simulink model "sampleModel1"  (R2021a)
settings: Solver=VariableStepAuto  StartTime=0.0  StopTime=50  RelTol=1e-3
undefined symbols (not defined in the file): DiscIntNeverNeededParam, magnitude, Newton, Raphson
libraries: simulink x92, pid_lib x10
(part 2 of 5)

== system sampleModel1/cfblk99 ==
  cfblk1 : Inport
  cfblk11 : Inport  Port=2
  cfblk12 : Inport  Port=3
  cfblk13 : Inport  Port=4
  cfblk14 : Inport  Port=5
  Action Port : ActionPort  ActionPortLabel=else
  cfblk10 : Subsystem
  cfblk3 : simulink/Math Operations/Slider Gain  gain=1  low=0  high=2
  cfblk4 : Squeeze
  cfblk5 : Sqrt  Operator=rSqrt  AlgorithmType=Newton-Raphson  SaturateOnIntegerOverflow=on
  cfblk6 : Constant  Value=[-6555592.349522]  SampleTime=1
  cfblk7 : Constant  Value=[-863944611.741175]  SampleTime=1
  cfblk8 : Constant  Value=[-802487376.058000]  SampleTime=1
  cfblk9 : Subsystem
  cfblk2 : Outport
  cfblk15 : Outport  Port=2
  wires:
  cfblk11/1 -> cfblk4/1
  cfblk12/1 -> cfblk5/1
  cfblk7/1 -> cfblk15/1
  cfblk3/1 -> cfblk10/1(cfblk1), cfblk9/4(cfblk10)
  cfblk1/1 -> cfblk10/2(cfblk10)
  cfblk4/1 -> cfblk3/1
  cfblk6/1 -> cfblk10/3(cfblk11)
  cfblk8/1 -> cfblk2/1
  cfblk5/1 -> cfblk10/4(cfblk12)
  cfblk14/1 -> cfblk9/1(cfblk1)
  cfblk13/1 -> cfblk10/5(cfblk13)
  cfblk10/1(cfblk2) -> cfblk9/2(cfblk8)
  cfblk10/2(cfblk14) -> cfblk9/3(cfblk9)

== system sampleModel1/cfblk101/cfblk12 ==
  cfblk1 : Inport
  cfblk6 : Inport  Port=2
  cfblk7 : Inport  Port=3
  cfblk3 : Delay
  cfblk4 : Product  Inputs=*
  cfblk5 : Constant  Value=[722696352.833129]  SampleTime=1
  cfblk2 : Outport
  cfblk8 : Outport  Port=2
  wires:
  cfblk7/1 -> cfblk8/1
  cfblk1/1 -> cfblk4/1
  cfblk4/1 -> cfblk3/1
  cfblk6/1 -> cfblk2/1

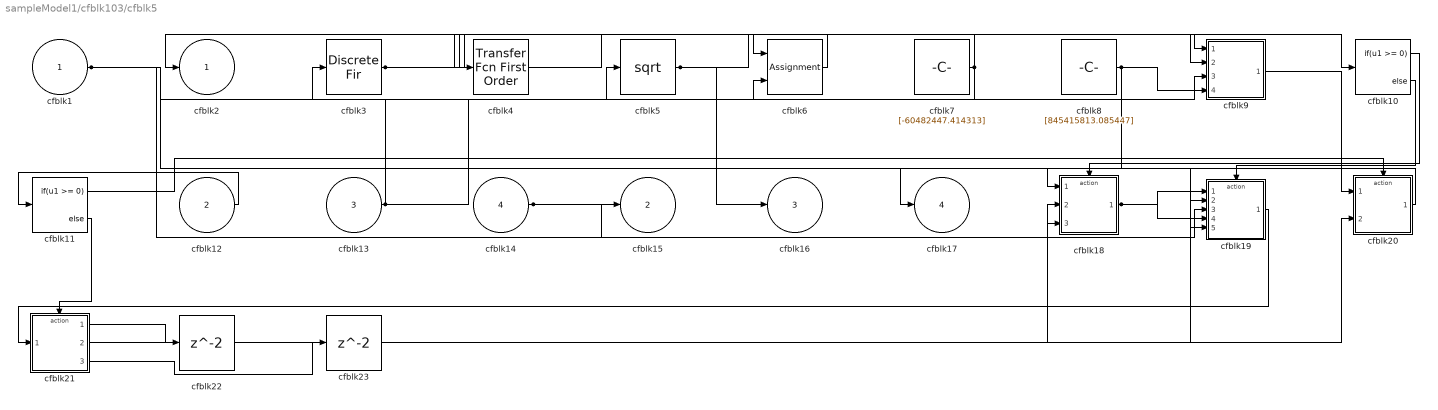
== system sampleModel1/cfblk103/cfblk5 ==
  cfblk1 : Inport
  cfblk12 : Inport  Port=2
  cfblk13 : Inport  Port=3
  cfblk14 : Inport  Port=4
  cfblk10 : If  IfExpression=u1 >= 0  SampleTime=1
  cfblk11 : If  IfExpression=u1 >= 0  SampleTime=1
  cfblk18 : Subsystem  TreatAsAtomicUnit=on
  cfblk19 : Subsystem  TreatAsAtomicUnit=on
  cfblk20 : Subsystem  TreatAsAtomicUnit=on
  cfblk21 : Subsystem  TreatAsAtomicUnit=on
  cfblk22 : Delay
  cfblk23 : Delay
  cfblk3 : DiscreteFir
  cfblk4 : simulink/Discrete/Transfer Fcn First Order  PoleZ=0.95  ICPrevOutput=0.0  DoSatur=off
  cfblk5 : Sqrt  SaturateOnIntegerOverflow=on
  cfblk6 : Assignment  DiagnosticForDimensions=Warning  IndexOptions=Index vector (dialog)  Indices=1  OutputSizes=1
  cfblk7 : Constant  Value=[-60482447.414313]  SampleTime=1
  cfblk8 : Constant  Value=[845415813.085447]  SampleTime=1
  cfblk9 : Subsystem
  cfblk2 : Outport
  cfblk15 : Outport  Port=2
  cfblk16 : Outport  Port=3
  cfblk17 : Outport  Port=4
  wires:
  cfblk20/1(cfblk2) -> cfblk17/1
  cfblk19/1(cfblk2) -> cfblk21/1(cfblk1)
  cfblk18/1(cfblk2) -> cfblk19/1(cfblk1), cfblk19/4(cfblk15)
  cfblk8/1 -> cfblk18/1(cfblk1), cfblk9/4(cfblk16)
  cfblk3/1 -> cfblk9/1(cfblk1), cfblk10/1
  cfblk14/1 -> cfblk15/1, cfblk19/3(cfblk14)
  cfblk13/1 -> cfblk5/1, cfblk3/1
  cfblk6/1 -> cfblk2/1
  cfblk4/1 -> cfblk6/1
  cfblk5/1 -> cfblk16/1, cfblk9/2(cfblk14)
  cfblk9/1(cfblk2) -> cfblk20/1(cfblk1)
  cfblk1/1 -> cfblk18/2(cfblk6), cfblk9/3(cfblk15), cfblk19/5(cfblk16)
  cfblk12/1 -> cfblk11/1
  cfblk21/2(cfblk14) -> cfblk20/2(cfblk11)
  cfblk7/1 -> cfblk4/1, cfblk6/2
  cfblk10/1 -> cfblk18/Action
  cfblk10/2 -> cfblk19/Action
  cfblk11/1 -> cfblk20/Action
  cfblk11/2 -> cfblk21/Action
  cfblk21/1(cfblk2) -> cfblk22/1
  cfblk22/1 -> cfblk19/2(cfblk13)
  cfblk21/3(cfblk15) -> cfblk23/1
  cfblk23/1 -> cfblk18/3(cfblk7)

== system sampleModel1/cfblk104/cfblk18 ==
  cfblk1 : Inport
  cfblk6 : Inport  Port=2
  cfblk7 : Inport  Port=3
  cfblk8 : Inport  Port=4
  Action Port : ActionPort  ActionPortLabel=if(u1 >= 0)
  cfblk10 : Subsystem  TreatAsAtomicUnit=on
  cfblk11 : Delay
  cfblk12 : Delay
  cfblk3 : pid_lib/PID Controller (2DOF)  Controller=PID  Form=Parallel  TimeDomain=Discrete-time  UseExternalTs=off  SampleTime=-1  IntegratorMethod=Forward Euler  FilterMethod=Forward Euler  ControllerParametersSource=internal  P=1  I=1  D=0  UseFilter=on  N=100  b=1  c=1  TunerSelectOption=Transfer Function Based (PID Tuner App)  InitialConditionSource=internal  InitialConditionForIntegrator=0  InitialConditionForFilter=0  DifferentiatorICPrevScaledInput=0  ExternalReset=none  TrackingMode=off  Kt=1  LimitOutput=off  SatLimitsSource=internal  UpperSaturationLimit=inf  LowerSaturationLimit=-inf  LinearizeAsGain=off  AntiWindupMode=none  Kb=1  POutMin=[]  POutMax=[]  IOutMin=[]  IOutMax=[]  DOutMin=[]  DOutMax=[]  NOutMin=[]  NOutMax=[]  bOutMin=[]  bOutMax=[]  cOutMin=[]  cOutMax=[]  SumOutMin=[]  SumOutMax=[]  SaturationOutMin=[]  SaturationOutMax=[]  PParamMin=[]  PParamMax=[]  IParamMin=[]  IParamMax=[]  DParamMin=[]  DParamMax=[]  NParamMin=[]  NParamMax=[]  bParamMin=[]  bParamMax=[]  cParamMin=[]  cParamMax=[]  KbParamMin=[]  KbParamMax=[]  KtParamMin=[]  KtParamMax=[]  KbOutMin=[]  KbOutMax=[]  KtOutMin=[]  KtOutMax=[]  IntegratorOutMin=[]  IntegratorOutMax=[]  FilterOutMin=[]  FilterOutMax=[]  SumI1OutMin=[]  SumI1OutMax=[]  SumI2OutMin=[]  SumI2OutMax=[]  SumI3OutMin=[]  SumI3OutMax=[]  SumI4OutMin=[]  SumI4OutMax=[]  SumDOutMin=[]  SumDOutMax=[]  Sum1OutMin=[]  Sum1OutMax=[]  Sum2OutMin=[]  Sum2OutMax=[]  Sum3OutMin=[]  Sum3OutMax=[]  DifferentiatorOutMin=[]  DifferentiatorOutMax=[]  FilterDiffOutCoefMin=[]  FilterDiffOutCoefMax=[]  ReciprocalOutMin=[]  ReciprocalOutMax=[]  SumDenOutMin=[]  SumDenOutMax=[]  SumNumOutMin=[]  SumNumOutMax=[]  DivideOutMin=[]  DivideOutMax=[]  UdiffTsProdOutMin=[]  UdiffTsProdOutMax=[]  NTsProdOutMin=[]  NTsProdOutMax=[]  UintegralTsProdOutMin=[]  UintegralTsProdOutMax=[]  UngainTsProdOutMin=[]  UngainTsProdOutMax=[]  IntegratorContinuousStateAttributes=''  IntegratorStateMustResolveToSignalObject=off  IntegratorRTWStateStorageClass=Auto  FilterContinuousStateAttributes=''  FilterStateMustResolveToSignalObject=off  FilterRTWStateStorageClass=Auto  ParallelPVariant=InternalParameters  IdealPVariant=Disabled  IVariant=InternalParameters  DVariant=InternalParameters  bVariant=InternalParameters  cVariant=InternalParameters  IntegratorVariant=Discrete  SatVariant=Disabled  AWVariant=Passthrough  PCopyVariant=Disabled  TRVariant=Disabled  FdbkBlocksVariant=Forward  IdealPFdbkVariant=Disabled  SatFdbkVariant=Disabled  DerivativeFilterVariant=ForwardEulerFilter  NVariant=InternalParameters  NCopyVariant=Disabled  FilterICVariant=InternalICsFilter  IntegratorICVariant=InternalICs  ExternalResetVariant=Disabled  TRSumVariant=Passthrough  SumFdbkVariant=Disabled  SumVariant=Sum_PID  TsampFilterVariant=InternalTs  TsampNgainVariant=Passthrough  TsampIntegralVariant=Passthrough  ExternalSaturationOutDataTypeStr=Inherit: Same as second input
      settings: SourceProductBaseCode=SL
  cfblk4 : Constant  Value=[-500662489.432987]  SampleTime=1
  cfblk5 : If  IfExpression=u1 >= 0  SampleTime=1
  cfblk9 : Subsystem  TreatAsAtomicUnit=on
  cfblk2 : Outport
  wires:
  cfblk8/1 -> cfblk3/1
  cfblk9/1(cfblk2) -> cfblk3/2
  cfblk7/1 -> cfblk10/1(cfblk1)
  cfblk6/1 -> cfblk2/1
  cfblk1/1 -> cfblk9/1(cfblk1)
  cfblk10/2(cfblk6) -> cfblk9/2(cfblk9)
  cfblk5/1 -> cfblk9/Action
  cfblk5/2 -> cfblk10/Action
  cfblk3/1 -> cfblk11/1
  cfblk11/1 -> cfblk9/3(cfblk10)
  cfblk10/1(cfblk2) -> cfblk12/1
  cfblk12/1 -> cfblk5/1

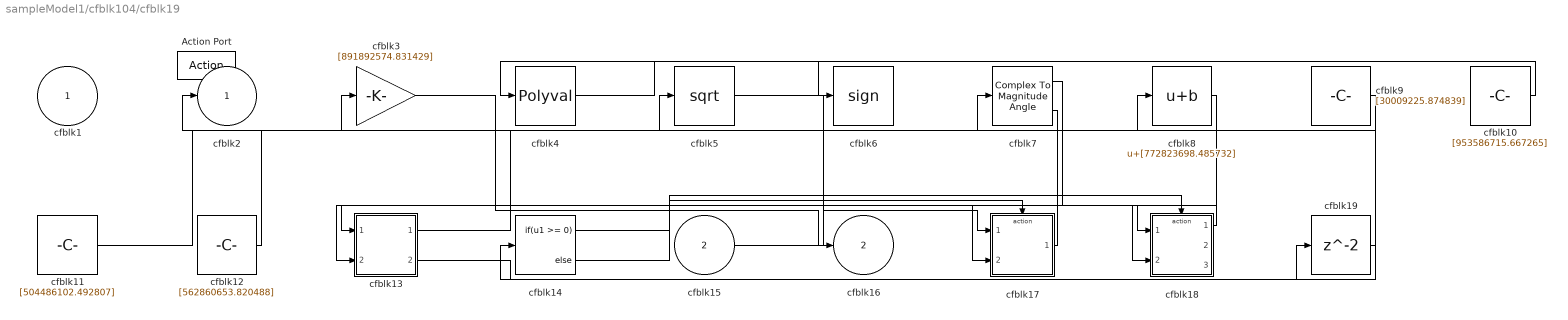
== system sampleModel1/cfblk104/cfblk19 ==
  cfblk1 : Inport
  cfblk15 : Inport  Port=2
  Action Port : ActionPort  ActionPortLabel=else
  cfblk10 : Constant  Value=[953586715.667265]  SampleTime=1
  cfblk11 : Constant  Value=[504486102.492807]  SampleTime=1
  cfblk12 : Constant  Value=[562860653.820488]  SampleTime=1
  cfblk13 : Subsystem
  cfblk14 : If  IfExpression=u1 >= 0  SampleTime=1
  cfblk17 : Subsystem  TreatAsAtomicUnit=on
  cfblk18 : Subsystem  TreatAsAtomicUnit=on
  cfblk19 : Delay
  cfblk3 : Gain  Gain=[891892574.831429]
  cfblk4 : Polyval  Coefs=[ +2.081618890e-019, -1.441693666e-014, +4.719686976e-010, -8.536869453e-006, +1.621573104e-001, -8.087801117e+001 ]
  cfblk5 : Sqrt  SaturateOnIntegerOverflow=on
  cfblk6 : Signum
  cfblk7 : ComplexToMagnitudeAngle
  cfblk8 : Bias  Bias=[772823698.485732]
  cfblk9 : Constant  Value=[30009225.874839]  SampleTime=1
  cfblk2 : Outport
  cfblk16 : Outport  Port=2
  wires:
  cfblk15/1 -> cfblk18/1(cfblk1)
  cfblk5/1 -> cfblk17/1(cfblk1)
  cfblk13/1(cfblk2) -> cfblk5/1
  cfblk9/1 -> cfblk14/1
  cfblk8/1 -> cfblk18/2(cfblk8)
  cfblk7/1 -> cfblk17/2(cfblk15)
  cfblk10/1 -> cfblk4/1
  cfblk12/1 -> cfblk2/1
  cfblk11/1 -> cfblk8/1
  cfblk3/1 -> cfblk16/1
  cfblk18/1(cfblk2) -> cfblk13/1(cfblk1)
  cfblk17/1(cfblk2) -> cfblk3/1
  cfblk4/1 -> cfblk6/1
  cfblk7/2 -> cfblk13/2(cfblk10)
  cfblk14/1 -> cfblk17/Action
  cfblk14/2 -> cfblk18/Action
  cfblk13/2(cfblk11) -> cfblk19/1
  cfblk19/1 -> cfblk7/1

== system sampleModel1/cfblk104/cfblk20 ==
  cfblk1 : Inport
  cfblk11 : Inport  Port=2
  cfblk12 : Inport  Port=3
  Action Port : ActionPort  ActionPortLabel=if(u1 >= 0)
  cfblk10 : Constant  Value=[940577982.224245]  SampleTime=1
  cfblk3 : DiscreteTransferFcn
  cfblk4 : DiscreteIntegrator  SampleTime=-1  ICPrevOutput=DiscIntNeverNeededParam  ICPrevScaledInput=DiscIntNeverNeededParam
  cfblk5 : Product  Inputs=*
  cfblk6 : Squeeze
  cfblk7 : Sqrt  SaturateOnIntegerOverflow=on
  cfblk8 : Constant  Value=[3734174.076073]  SampleTime=1
  cfblk9 : Constant  Value=[-760670117.794091]  SampleTime=1
  cfblk2 : Outport
  wires:
  cfblk1/1 -> cfblk5/1
  cfblk4/1 -> cfblk2/1
  cfblk10/1 -> cfblk3/1
  cfblk9/1 -> cfblk4/1
  cfblk8/1 -> cfblk7/1
  cfblk12/1 -> cfblk6/1

== system sampleModel1/cfblk104/cfblk21 ==
  cfblk1 : Inport
  cfblk9 : Inport  Port=2
  Action Port : ActionPort  ActionPortLabel=else
  cfblk11 : Subsystem  TreatAsAtomicUnit=on
  cfblk12 : Subsystem  TreatAsAtomicUnit=on
  cfblk13 : Delay
  cfblk14 : Delay
  cfblk3 : Assignment  DiagnosticForDimensions=Warning  IndexOptions=Index vector (dialog)  Indices=1  OutputSizes=1
  cfblk4 : Sin  TimeSource=Use external signal  SampleTime=0
  cfblk5 : simulink/Math Operations/Slider Gain  gain=1  low=0  high=2
  cfblk6 : Squeeze
  cfblk7 : Constant  Value=[516497574.355924]  SampleTime=1
  cfblk8 : If  IfExpression=u1 >= 0  SampleTime=1
  cfblk2 : Outport
  cfblk10 : Outport  Port=2
  wires:
  cfblk9/1 -> cfblk2/1
  cfblk7/1 -> cfblk5/1
  cfblk5/1 -> cfblk4/1
  cfblk4/1 -> cfblk3/1
  cfblk11/1(cfblk2) -> cfblk6/1
  cfblk11/2(cfblk14) -> cfblk3/2
  cfblk12/1(cfblk2) -> cfblk11/2(cfblk13)
  cfblk12/2(cfblk10) -> cfblk10/1
  cfblk1/1 -> cfblk12/1(cfblk1)
  cfblk8/1 -> cfblk11/Action
  cfblk8/2 -> cfblk12/Action
  cfblk6/1 -> cfblk13/1
  cfblk13/1 -> cfblk11/1(cfblk1)
  cfblk3/1 -> cfblk14/1
  cfblk14/1 -> cfblk8/1

== system sampleModel1/cfblk105/cfblk6 ==
  cfblk1 : Inport
  cfblk10 : Subsystem  TreatAsAtomicUnit=on
  cfblk11 : Delay
  cfblk3 : Reshape
  cfblk4 : Assignment  DiagnosticForDimensions=Warning  IndexOptions=Index vector (dialog)  Indices=1  OutputSizes=1
  cfblk5 : Constant  Value=[255394404.156732]  SampleTime=1
  cfblk6 : Constant  Value=[553929380.128672]  SampleTime=1
  cfblk7 : If  IfExpression=u1 >= 0  SampleTime=1
  cfblk9 : Subsystem  TreatAsAtomicUnit=on
  cfblk2 : Outport
  cfblk8 : Outport  Port=2
  wires:
  cfblk6/1 -> cfblk4/1
  cfblk3/1 -> cfblk4/2
  cfblk10/1(cfblk2) -> cfblk9/1(cfblk1)
  cfblk4/1 -> cfblk10/1(cfblk1)
  cfblk10/2(cfblk13) -> cfblk2/1, cfblk9/2(cfblk8)
  cfblk5/1 -> cfblk8/1, cfblk3/1
  cfblk1/1 -> cfblk10/2(cfblk12)
  cfblk7/1 -> cfblk9/Action
  cfblk7/2 -> cfblk10/Action
  cfblk9/1(cfblk2) -> cfblk11/1
  cfblk11/1 -> cfblk7/1

== system sampleModel1/cfblk107/cfblk17 ==
  cfblk1 : Inport
  Action Port : ActionPort  ActionPortLabel=if(u1 >= 0)
  cfblk3 : Gain  Gain=[234365118.944540]
  cfblk4 : simulink/Math Operations/Slider Gain  gain=1  low=0  high=2
  cfblk5 : Math  Operator=magnitude^2  SaturateOnIntegerOverflow=on
  cfblk6 : Bias  Bias=[-274123626.763380]
  cfblk7 : Constant  Value=[-863023427.250108]  SampleTime=1
  cfblk9 : Delay
  cfblk2 : Outport
  cfblk8 : Outport  Port=2
  wires:
  cfblk1/1 -> cfblk4/1
  cfblk4/1 -> cfblk8/1
  cfblk7/1 -> cfblk2/1
  cfblk5/1 -> cfblk6/1, cfblk3/1
  cfblk6/1 -> cfblk9/1
  cfblk9/1 -> cfblk5/1

== system sampleModel1/cfblk107/cfblk18 ==
  cfblk1 : Inport
  cfblk6 : Inport  Port=2
  cfblk7 : Inport  Port=3
  Action Port : ActionPort  ActionPortLabel=else
  cfblk3 : simulink/Discrete/Tapped Delay  vinit=0.0  samptime=-1  NumDelays=1  DelayOrder=Oldest  includeCurrent=off
  cfblk4 : Constant  Value=[319233537.523609]  SampleTime=1
  cfblk5 : Constant  Value=[609478027.625537]  SampleTime=1
  cfblk2 : Outport
  wires:
  cfblk5/1 -> cfblk3/1
  cfblk3/1 -> cfblk2/1

== system sampleModel1/cfblk108/cfblk9 ==
  cfblk1 : Inport
  cfblk8 : Inport  Port=2
  cfblk9 : Inport  Port=3
  cfblk3 : Sum  Inputs=+
  cfblk4 : Sum  Inputs=+-
  cfblk5 : Constant  Value=[194121577.220702]  SampleTime=1
  cfblk6 : Constant  Value=[830027987.513452]  SampleTime=1
  cfblk7 : Subsystem
  cfblk2 : Outport
  cfblk10 : Outport  Port=2
  wires:
  cfblk6/1 -> cfblk10/1
  cfblk9/1 -> cfblk2/1
  cfblk1/1 -> cfblk4/1
  cfblk8/1 -> cfblk3/1
  cfblk4/1 -> cfblk7/1(cfblk1)
  cfblk3/1 -> cfblk4/2

== system sampleModel1/cfblk109/cfblk10 ==
  cfblk1 : Inport
  cfblk13 : Inport  Port=2
  cfblk14 : Inport  Port=3
  cfblk15 : Inport  Port=4
  cfblk10 : Constant  Value=[-175853444.571278]  SampleTime=1
  cfblk11 : Constant  Value=[46253064.780772]  SampleTime=1
  cfblk12 : Subsystem
  cfblk3 : UnitDelay  SampleTime=-1  HasFrameUpgradeWarning=on
  cfblk4 : DotProduct  InputSameDT=on  OutDataTypeStr=Inherit: Inherit via internal rule
  cfblk5 : UnaryMinus
  cfblk6 : Product
  cfblk7 : simulink/Math Operations/Slider Gain  gain=1  low=0  high=2
  cfblk8 : Constant  Value=[-372396158.254895]  SampleTime=1
  cfblk9 : Constant  Value=[-911852416.361733]  SampleTime=1
  cfblk2 : Outport
  cfblk16 : Outport  Port=2
  wires:
  cfblk7/1 -> cfblk6/1
  cfblk14/1 -> cfblk2/1
  cfblk13/1 -> cfblk7/1
  cfblk1/1 -> cfblk6/2
  cfblk8/1 -> cfblk16/1
  cfblk4/1 -> cfblk5/1
  cfblk15/1 -> cfblk12/1(cfblk1)
  cfblk11/1 -> cfblk4/1
  cfblk10/1 -> cfblk3/1
  cfblk6/1 -> cfblk4/2

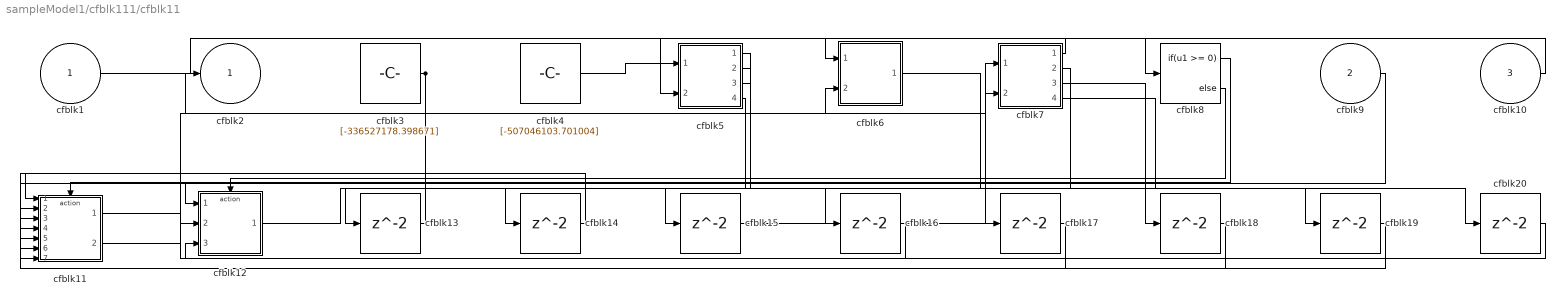
== system sampleModel1/cfblk111/cfblk11 ==
  cfblk1 : Inport
  cfblk9 : Inport  Port=2
  cfblk10 : Inport  Port=3
  cfblk11 : Subsystem  TreatAsAtomicUnit=on
  cfblk12 : Subsystem  TreatAsAtomicUnit=on
  cfblk{13..20} (8 alike) : Delay
  cfblk3 : Constant  Value=[-336527178.398671]  SampleTime=1
  cfblk4 : Constant  Value=[-507046103.701004]  SampleTime=1
  cfblk5 : Subsystem
  cfblk6 : Subsystem
  cfblk7 : Subsystem
  cfblk8 : If  IfExpression=u1 >= 0  SampleTime=1
  cfblk2 : Outport
  wires:
  cfblk4/1 -> cfblk5/1(cfblk1)
  cfblk9/1 -> cfblk12/1(cfblk1)
  cfblk1/1 -> cfblk8/1
  cfblk11/1(cfblk2) -> cfblk7/1(cfblk1)
  cfblk10/1 -> cfblk6/1(cfblk1)
  cfblk7/1(cfblk2) -> cfblk5/2(cfblk12)
  cfblk5/3(cfblk14) -> cfblk2/1
  cfblk11/2(cfblk16) -> cfblk6/2(cfblk7)
  cfblk3/1 -> cfblk11/3(cfblk11), cfblk11/7(cfblk15)
  cfblk8/1 -> cfblk11/Action
  cfblk8/2 -> cfblk12/Action
  cfblk5/1(cfblk2) -> cfblk13/1
  cfblk13/1 -> cfblk11/1(cfblk1)
  cfblk5/2(cfblk13) -> cfblk14/1
  cfblk14/1 -> cfblk11/2(cfblk10)
  cfblk5/4(cfblk15) -> cfblk15/1
  cfblk15/1 -> cfblk7/2(cfblk14)
  cfblk7/2(cfblk15) -> cfblk16/1
  cfblk16/1 -> cfblk12/3(cfblk11)
  cfblk12/1(cfblk2) -> cfblk17/1
  cfblk17/1 -> cfblk11/5(cfblk13)
  cfblk7/3(cfblk16) -> cfblk18/1
  cfblk18/1 -> cfblk11/4(cfblk12)
  cfblk7/4(cfblk17) -> cfblk19/1
  cfblk19/1 -> cfblk11/6(cfblk14)
  cfblk6/1(cfblk2) -> cfblk20/1
  cfblk20/1 -> cfblk12/2(cfblk10)

== system sampleModel1/cfblk111/cfblk16 ==
  cfblk1 : Inport
  cfblk6 : Inport  Port=2
  Action Port : ActionPort  ActionPortLabel=if(u1 >= 0)
  cfblk3 : Math  Operator=mod  SaturateOnIntegerOverflow=on
  cfblk4 : Constant  Value=[416678460.223587]  SampleTime=1
  cfblk5 : Constant  Value=[-246012607.536982]  SampleTime=1
  cfblk2 : Outport
  cfblk7 : Outport  Port=2
  wires:
  cfblk4/1 -> cfblk3/1
  cfblk3/1 -> cfblk2/1
  cfblk5/1 -> cfblk3/2
  cfblk6/1 -> cfblk7/1

== system sampleModel1/cfblk111/cfblk17 ==
  cfblk1 : Inport
  cfblk13 : Inport  Port=2
  Action Port : ActionPort  ActionPortLabel=else
  cfblk10 : UnaryMinus
  cfblk11 : simulink/Math Operations/Slider Gain  gain=1  low=0  high=2
  cfblk12 : Constant  Value=[-711731510.920077]  SampleTime=1
  cfblk17 : Delay
  cfblk3 : UnitDelay  SampleTime=-1  HasFrameUpgradeWarning=on
  cfblk4 : Abs
  cfblk5 : Bias  Bias=[158723366.272055]
  cfblk6 : Bias  Bias=[242313084.935745]
  cfblk7 : Sum  Inputs=+-
  cfblk8 : Product  Inputs=**
  cfblk9 : Trigonometry
  cfblk2 : Outport
  cfblk14 : Outport  Port=2
  cfblk15 : Outport  Port=3
  cfblk16 : Outport  Port=4
  wires:
  cfblk10/1 -> cfblk14/1
  cfblk13/1 -> cfblk7/1
  cfblk4/1 -> cfblk9/1
  cfblk5/1 -> cfblk10/1, cfblk6/1
  cfblk12/1 -> cfblk11/1
  cfblk11/1 -> cfblk4/1
  cfblk1/1 -> cfblk8/1, cfblk2/1
  cfblk9/1 -> cfblk3/1
  cfblk8/1 -> cfblk7/2
  cfblk3/1 -> cfblk15/1, cfblk5/1
  cfblk6/1 -> cfblk16/1
  cfblk7/1 -> cfblk17/1
  cfblk17/1 -> cfblk8/2

== system sampleModel1/cfblk112/cfblk11 ==
  cfblk1 : Inport
  cfblk12 : Inport  Port=2
  Action Port : ActionPort  ActionPortLabel=if(u1 >= 0)
  cfblk10 : Constant  Value=[-370015826.295377]  SampleTime=1
  cfblk11 : If  IfExpression=u1 >= 0  SampleTime=1
  cfblk13 : Subsystem  TreatAsAtomicUnit=on
  cfblk14 : Subsystem  TreatAsAtomicUnit=on
  cfblk15 : Delay
  cfblk3 : UnaryMinus
  cfblk4 : simulink/Math Operations/Slider Gain  gain=1  low=0  high=2
  cfblk5 : Sqrt  Operator=rSqrt  AlgorithmType=Newton-Raphson  SaturateOnIntegerOverflow=on
  cfblk6 : Trigonometry
  cfblk7 : UnaryMinus
  cfblk8 : Constant  Value=[802430284.434058]  SampleTime=1
  cfblk9 : Constant  Value=[-33439961.092707]  SampleTime=1
  cfblk2 : Outport
  wires:
  cfblk4/1 -> cfblk14/1(cfblk1)
  cfblk10/1 -> cfblk6/1
  cfblk9/1 -> cfblk7/1
  cfblk7/1 -> cfblk3/1
  cfblk14/1(cfblk2) -> cfblk13/1(cfblk1)
  cfblk6/1 -> cfblk5/1
  cfblk5/1 -> cfblk11/1
  cfblk1/1 -> cfblk4/1
  cfblk12/1 -> cfblk2/1
  cfblk14/2(cfblk13) -> cfblk13/2(cfblk13)
  cfblk3/1 -> cfblk14/2(cfblk11)
  cfblk11/1 -> cfblk13/Action
  cfblk11/2 -> cfblk14/Action
  cfblk13/1(cfblk2) -> cfblk15/1
  cfblk15/1 -> cfblk14/3(cfblk12)

== system sampleModel1/cfblk112/cfblk12 ==
  cfblk1 : Inport
  cfblk9 : Inport  Port=2
  cfblk10 : Inport  Port=3
  Action Port : ActionPort  ActionPortLabel=else
  cfblk11 : Delay
  cfblk3 : DiscreteStateSpace  SampleTime=-1
  cfblk4 : Product  Inputs=*
  cfblk5 : Product
  cfblk6 : Reshape
  cfblk7 : Constant  Value=[293128861.832892]  SampleTime=1
  cfblk8 : Subsystem
  cfblk2 : Outport
  wires:
  cfblk7/1 -> cfblk2/1
  cfblk6/1 -> cfblk5/1
  cfblk4/1 -> cfblk5/2
  cfblk1/1 -> cfblk3/1
  cfblk9/1 -> cfblk6/1
  cfblk10/1 -> cfblk8/1(cfblk1)
  cfblk5/1 -> cfblk11/1
  cfblk11/1 -> cfblk4/1

== system sampleModel1/cfblk114/cfblk11 ==
  cfblk1 : Inport
  cfblk13 : Inport  Port=2
  cfblk14 : Inport  Port=3
  cfblk10 : Constant  Value=[-274061940.097837]  SampleTime=1
  cfblk11 : Constant  Value=[854560708.798719]  SampleTime=1
  cfblk12 : Subsystem
  cfblk18 : Delay
  cfblk3 : DotProduct  InputSameDT=on  OutDataTypeStr=Inherit: Inherit via internal rule
  cfblk4 : ComplexToRealImag
  cfblk5 : Signum
  cfblk6 : Sqrt  SaturateOnIntegerOverflow=on
  cfblk7 : Constant  Value=[92027810.090725]  SampleTime=1
  cfblk8 : Constant  Value=[373524938.370021]  SampleTime=1
  cfblk9 : Constant  Value=[145197070.152737]  SampleTime=1
  cfblk2 : Outport
  cfblk15 : Outport  Port=2
  cfblk16 : Outport  Port=3
  cfblk17 : Outport  Port=4
  wires:
  cfblk8/1 -> cfblk4/1
  cfblk13/1 -> cfblk6/1
  cfblk5/1 -> cfblk2/1
  cfblk4/1 -> cfblk5/1
  cfblk4/2 -> cfblk16/1
  cfblk6/1 -> cfblk3/1
  cfblk12/1(cfblk2) -> cfblk3/2
  cfblk11/1 -> cfblk15/1
  cfblk7/1 -> cfblk17/1
  cfblk14/1 -> cfblk12/1(cfblk1)
  cfblk9/1 -> cfblk12/2(cfblk10)
  cfblk10/1 -> cfblk12/3(cfblk11)
  cfblk1/1 -> cfblk12/4(cfblk12), cfblk12/6(cfblk14)
  cfblk3/1 -> cfblk18/1
  cfblk18/1 -> cfblk12/5(cfblk13)

== system sampleModel1/cfblk115/cfblk12 ==
  cfblk1 : Inport
  cfblk9 : Inport  Port=2
  cfblk10 : Inport  Port=3
  cfblk3 : simulink/Discrete/Tapped Delay  vinit=0.0  samptime=-1  NumDelays=1  DelayOrder=Oldest  includeCurrent=off
  cfblk4 : ComplexToRealImag
  cfblk5 : PermuteDimensions
  cfblk6 : Constant  Value=[776999277.993085]  SampleTime=1
  cfblk7 : Constant  Value=[879343192.545425]  SampleTime=1
  cfblk8 : Constant  Value=[-122389967.939899]  SampleTime=1
  cfblk2 : Outport
  wires:
  cfblk8/1 -> cfblk2/1
  cfblk3/1 -> cfblk5/1
  cfblk1/1 -> cfblk3/1
  cfblk9/1 -> cfblk4/1

== system sampleModel1/cfblk115/cfblk14 ==
  cfblk1 : Inport
  cfblk11 : Inport  Port=2
  Action Port : ActionPort  ActionPortLabel=if(u1 >= 0)
  cfblk10 : If  IfExpression=u1 >= 0  SampleTime=1
  cfblk13 : Subsystem  TreatAsAtomicUnit=on
  cfblk14 : Subsystem  TreatAsAtomicUnit=on
  cfblk{15..19} (5 alike) : Delay
  cfblk3 : Product  Inputs=*
  cfblk4 : Constant  Value=[-489992420.979216]  SampleTime=1
  cfblk5 : Constant  Value=[178204759.844577]  SampleTime=1
  cfblk6 : Constant  Value=[176026825.316252]  SampleTime=1
  cfblk7 : Subsystem
  cfblk8 : Subsystem
  cfblk9 : Subsystem
  cfblk2 : Outport
  cfblk12 : Outport  Port=2
  wires:
  cfblk5/1 -> cfblk3/1
  cfblk9/1(cfblk2) -> cfblk8/1(cfblk1)
  cfblk14/1(cfblk2) -> cfblk12/1
  cfblk3/1 -> cfblk8/2(cfblk12)
  cfblk1/1 -> cfblk10/1
  cfblk6/1 -> cfblk2/1
  cfblk11/1 -> cfblk7/2(cfblk10)
  cfblk13/1(cfblk2) -> cfblk9/1(cfblk1)
  cfblk13/2(cfblk8) -> cfblk9/2(cfblk12)
  cfblk8/2(cfblk13) -> cfblk7/3(cfblk11)
  cfblk10/1 -> cfblk13/Action
  cfblk10/2 -> cfblk14/Action
  cfblk8/1(cfblk2) -> cfblk15/1
  cfblk15/1 -> cfblk13/1(cfblk1)
  cfblk7/1(cfblk2) -> cfblk16/1
  cfblk16/1 -> cfblk9/3(cfblk13)
  cfblk7/2(cfblk12) -> cfblk17/1
  cfblk17/1 -> cfblk14/2(cfblk11)
  cfblk14/2(cfblk12) -> cfblk18/1
  cfblk18/1 -> cfblk7/1(cfblk1)
  cfblk9/2(cfblk14) -> cfblk19/1
  cfblk19/1 -> cfblk14/1(cfblk1)

== system sampleModel1/cfblk115/cfblk15 ==
  cfblk1 : Inport
  cfblk9 : Inport  Port=2
  cfblk10 : Inport  Port=3
  Action Port : ActionPort  ActionPortLabel=else
  cfblk3 : simulink/Math Operations/Slider Gain  gain=1  low=0  high=2
  cfblk4 : Sqrt  Operator=rSqrt  AlgorithmType=Newton-Raphson  SaturateOnIntegerOverflow=on
  cfblk5 : Abs
  cfblk6 : Signum
  cfblk7 : Abs
  cfblk8 : Constant  Value=[-136387865.048140]  SampleTime=1
  cfblk2 : Outport
  wires:
  cfblk3/1 -> cfblk5/1
  cfblk5/1 -> cfblk6/1
  cfblk4/1 -> cfblk7/1
  cfblk7/1 -> cfblk3/1
  cfblk8/1 -> cfblk2/1
  cfblk1/1 -> cfblk4/1

== system sampleModel1/cfblk73/cfblk17 ==
  cfblk1 : Inport
  cfblk5 : Inport  Port=2
  cfblk6 : Inport  Port=3
  Action Port : ActionPort  ActionPortLabel=if(u1 >= 0)
  cfblk3 : Math  Operator=log  SaturateOnIntegerOverflow=on
  cfblk4 : Signum
  cfblk2 : Outport
  cfblk7 : Outport  Port=2
  wires:
  cfblk1/1 -> cfblk4/1
  cfblk5/1 -> cfblk3/1
  cfblk6/1 -> cfblk7/1
  cfblk4/1 -> cfblk2/1

== system sampleModel1/cfblk73/cfblk18 ==
  cfblk1 : Inport
  cfblk9 : Inport  Port=2
  Action Port : ActionPort  ActionPortLabel=else
  cfblk11 : Subsystem  TreatAsAtomicUnit=on
  cfblk12 : Subsystem  TreatAsAtomicUnit=on
  cfblk13 : Delay
  cfblk3 : simulink/Discrete/Transfer Fcn Real Zero  ZeroZ=0.75  ICPrevInput=0.0  DoSatur=off
      settings: SourceProductBaseCode=SL
  cfblk4 : Sqrt  SaturateOnIntegerOverflow=on
  cfblk5 : Constant  Value=[153443031.229370]  SampleTime=1
  cfblk6 : Constant  Value=[-520135978.862565]  SampleTime=1
  cfblk7 : Constant  Value=[-942651695.071788]  SampleTime=1
  cfblk8 : If  IfExpression=u1 >= 0  SampleTime=1
  cfblk2 : Outport
  cfblk10 : Outport  Port=2
  wires:
  cfblk6/1 -> cfblk4/1
  cfblk9/1 -> cfblk11/1(cfblk1)
  cfblk3/1 -> cfblk2/1
  cfblk1/1 -> cfblk8/1
  cfblk5/1 -> cfblk11/2(cfblk16)
  cfblk4/1 -> cfblk3/1
  cfblk11/1(cfblk2) -> cfblk12/1(cfblk1)
  cfblk12/2(cfblk7) -> cfblk10/1
  cfblk7/1 -> cfblk12/2(cfblk6)
  cfblk8/1 -> cfblk11/Action
  cfblk8/2 -> cfblk12/Action
  cfblk12/1(cfblk2) -> cfblk13/1
  cfblk13/1 -> cfblk11/3(cfblk17)

== system sampleModel1/cfblk89/cfblk11 ==
  cfblk1 : Inport
  cfblk11 : Inport  Port=2
  cfblk10 : If  IfExpression=u1 >= 0  SampleTime=1
  cfblk13 : Subsystem  TreatAsAtomicUnit=on
  cfblk14 : Subsystem  TreatAsAtomicUnit=on
  cfblk3 : simulink/Math Operations/Slider Gain  gain=1  low=0  high=2
  cfblk4 : simulink/Math Operations/MinMax Running Resettable  Function=min  vinit=0.0
  cfblk5 : Rounding
  cfblk6 : Assignment  DiagnosticForDimensions=Warning  IndexOptions=Index vector (dialog)  Indices=1  OutputSizes=1
  cfblk7 : Constant  Value=[867519696.770665]  SampleTime=1
  cfblk8 : Constant  Value=[-467642322.184722]  SampleTime=1
  cfblk9 : Constant  Value=[-24792449.132153]  SampleTime=1
  cfblk2 : Outport
  cfblk12 : Outport  Port=2
  wires:
  cfblk1/1 -> cfblk5/1, cfblk14/3(cfblk7)
  cfblk8/1 -> cfblk13/1(cfblk1)
  cfblk14/1(cfblk2) -> cfblk4/1
  cfblk11/1 -> cfblk3/1
  cfblk6/1 -> cfblk12/1
  cfblk3/1 -> cfblk2/1
  cfblk5/1 -> cfblk10/1, cfblk14/4(cfblk8)
  cfblk7/1 -> cfblk13/2(cfblk10)
  cfblk13/1(cfblk2) -> cfblk14/1(cfblk1)
  cfblk4/1 -> cfblk6/1
  cfblk9/1 -> cfblk14/2(cfblk6)
  cfblk14/2(cfblk9) -> cfblk4/2
  cfblk14/3(cfblk10) -> cfblk6/2
  cfblk10/1 -> cfblk13/Action
  cfblk10/2 -> cfblk14/Action

== system sampleModel1/cfblk91/cfblk16 ==
  cfblk1 : Inport
  cfblk12 : Inport  Port=2
  cfblk13 : Inport  Port=3
  Action Port : ActionPort  ActionPortLabel=if(u1 >= 0)
  cfblk10 : Constant  Value=[320875932.625204]  SampleTime=1
  cfblk11 : If  IfExpression=u1 >= 0  SampleTime=1
  cfblk16 : Subsystem  TreatAsAtomicUnit=on
  cfblk17 : Subsystem  TreatAsAtomicUnit=on
  cfblk18 : Delay
  cfblk19 : Delay
  cfblk3 : UnaryMinus
  cfblk4 : Sum  Inputs=+-
  cfblk5 : Sin  TimeSource=Use external signal  SampleTime=0
  cfblk6 : Constant  Value=[-936154740.992043]  SampleTime=1
  cfblk7 : Constant  Value=[325307668.574429]  SampleTime=1
  cfblk8 : Constant  Value=[-539233865.365072]  SampleTime=1
  cfblk9 : Constant  Value=[249145833.986617]  SampleTime=1
  cfblk2 : Outport
  cfblk14 : Outport  Port=2
  cfblk15 : Outport  Port=3
  wires:
  cfblk16/1(cfblk2) -> cfblk5/1, cfblk19/1
  cfblk6/1 -> cfblk11/1
  cfblk3/1 -> cfblk4/1
  cfblk1/1 -> cfblk3/1
  cfblk7/1 -> cfblk14/1
  cfblk9/1 -> cfblk4/2, cfblk17/3(cfblk11)
  cfblk10/1 -> cfblk2/1
  cfblk4/1 -> cfblk17/2(cfblk10)
  cfblk8/1 -> cfblk16/1(cfblk1)
  cfblk12/1 -> cfblk15/1
  cfblk13/1 -> cfblk16/2(cfblk10)
  cfblk17/1(cfblk2) -> cfblk16/3(cfblk11)
  cfblk11/1 -> cfblk16/Action
  cfblk11/2 -> cfblk17/Action
  cfblk5/1 -> cfblk18/1
  cfblk18/1 -> cfblk17/1(cfblk1)
  cfblk19/1 -> cfblk17/4(cfblk12)

== system sampleModel1/cfblk91/cfblk17 ==
  cfblk1 : Inport
  Action Port : ActionPort  ActionPortLabel=else
  cfblk3 : Abs
  cfblk4 : UnaryMinus
  cfblk5 : simulink/Math Operations/MinMax Running Resettable  Function=min  vinit=0.0
  cfblk6 : Constant  Value=[923117146.207326]  SampleTime=1
  cfblk7 : Constant  Value=[-985302677.794306]  SampleTime=1
  cfblk8 : Constant  Value=[411901508.497767]  SampleTime=1
  cfblk9 : Constant  Value=[104619689.015460]  SampleTime=1
  cfblk2 : Outport
  wires:
  cfblk3/1 -> cfblk5/1
  cfblk9/1 -> cfblk3/1
  cfblk6/1 -> cfblk5/2
  cfblk7/1 -> cfblk2/1
  cfblk8/1 -> cfblk4/1

== system sampleModel1/cfblk91/cfblk18 ==
  cfblk1 : Inport
  cfblk12 : Inport  Port=2
  Action Port : ActionPort  ActionPortLabel=if(u1 >= 0)
  cfblk10 : Constant  Value=[456523695.645668]  SampleTime=1
  cfblk11 : If  IfExpression=u1 >= 0  SampleTime=1
  cfblk14 : Subsystem  TreatAsAtomicUnit=on
  cfblk15 : Subsystem  TreatAsAtomicUnit=on
  cfblk16 : Delay
  cfblk17 : Delay
  cfblk18 : Delay
  cfblk3 : pid_lib/PID Controller (2DOF)  Controller=PID  Form=Parallel  TimeDomain=Discrete-time  UseExternalTs=off  SampleTime=-1  IntegratorMethod=Forward Euler  FilterMethod=Forward Euler  ControllerParametersSource=internal  P=1  I=1  D=0  UseFilter=on  N=100  b=1  c=1  TunerSelectOption=Transfer Function Based (PID Tuner App)  InitialConditionSource=internal  InitialConditionForIntegrator=0  InitialConditionForFilter=0  DifferentiatorICPrevScaledInput=0  ExternalReset=none  TrackingMode=off  Kt=1  LimitOutput=off  SatLimitsSource=internal  UpperSaturationLimit=inf  LowerSaturationLimit=-inf  LinearizeAsGain=off  AntiWindupMode=none  Kb=1  POutMin=[]  POutMax=[]  IOutMin=[]  IOutMax=[]  DOutMin=[]  DOutMax=[]  NOutMin=[]  NOutMax=[]  bOutMin=[]  bOutMax=[]  cOutMin=[]  cOutMax=[]  SumOutMin=[]  SumOutMax=[]  SaturationOutMin=[]  SaturationOutMax=[]  PParamMin=[]  PParamMax=[]  IParamMin=[]  IParamMax=[]  DParamMin=[]  DParamMax=[]  NParamMin=[]  NParamMax=[]  bParamMin=[]  bParamMax=[]  cParamMin=[]  cParamMax=[]  KbParamMin=[]  KbParamMax=[]  KtParamMin=[]  KtParamMax=[]  KbOutMin=[]  KbOutMax=[]  KtOutMin=[]  KtOutMax=[]  IntegratorOutMin=[]  IntegratorOutMax=[]  FilterOutMin=[]  FilterOutMax=[]  SumI1OutMin=[]  SumI1OutMax=[]  SumI2OutMin=[]  SumI2OutMax=[]  SumI3OutMin=[]  SumI3OutMax=[]  SumI4OutMin=[]  SumI4OutMax=[]  SumDOutMin=[]  SumDOutMax=[]  Sum1OutMin=[]  Sum1OutMax=[]  Sum2OutMin=[]  Sum2OutMax=[]  Sum3OutMin=[]  Sum3OutMax=[]  DifferentiatorOutMin=[]  DifferentiatorOutMax=[]  FilterDiffOutCoefMin=[]  FilterDiffOutCoefMax=[]  ReciprocalOutMin=[]  ReciprocalOutMax=[]  SumDenOutMin=[]  SumDenOutMax=[]  SumNumOutMin=[]  SumNumOutMax=[]  DivideOutMin=[]  DivideOutMax=[]  UdiffTsProdOutMin=[]  UdiffTsProdOutMax=[]  NTsProdOutMin=[]  NTsProdOutMax=[]  UintegralTsProdOutMin=[]  UintegralTsProdOutMax=[]  UngainTsProdOutMin=[]  UngainTsProdOutMax=[]  IntegratorContinuousStateAttributes=''  IntegratorStateMustResolveToSignalObject=off  IntegratorRTWStateStorageClass=Auto  FilterContinuousStateAttributes=''  FilterStateMustResolveToSignalObject=off  FilterRTWStateStorageClass=Auto  ParallelPVariant=InternalParameters  IdealPVariant=Disabled  IVariant=InternalParameters  DVariant=InternalParameters  bVariant=InternalParameters  cVariant=InternalParameters  IntegratorVariant=Discrete  SatVariant=Disabled  AWVariant=Passthrough  PCopyVariant=Disabled  TRVariant=Disabled  FdbkBlocksVariant=Forward  IdealPFdbkVariant=Disabled  SatFdbkVariant=Disabled  DerivativeFilterVariant=ForwardEulerFilter  NVariant=InternalParameters  NCopyVariant=Disabled  FilterICVariant=InternalICsFilter  IntegratorICVariant=InternalICs  ExternalResetVariant=Disabled  TRSumVariant=Passthrough  SumFdbkVariant=Disabled  SumVariant=Sum_PID  TsampFilterVariant=InternalTs  TsampNgainVariant=Passthrough  TsampIntegralVariant=Passthrough  ExternalSaturationOutDataTypeStr=Inherit: Same as second input
      settings: SourceProductBaseCode=SL
  cfblk4 : Product  Inputs=*
  cfblk5 : Sum  Inputs=+-
  cfblk6 : Product  Inputs=*
  cfblk7 : DotProduct  InputSameDT=on  OutDataTypeStr=Inherit: Inherit via internal rule
  cfblk8 : DotProduct  InputSameDT=on  OutDataTypeStr=Inherit: Inherit via internal rule
  cfblk9 : Constant  Value=[871322751.033200]  SampleTime=1
  cfblk2 : Outport
  cfblk13 : Outport  Port=2
  wires:
  cfblk6/1 -> cfblk8/1
  cfblk8/1 -> cfblk4/1
  cfblk3/1 -> cfblk15/1(cfblk1)
  cfblk14/1(cfblk2) -> cfblk7/1, cfblk5/2
  cfblk10/1 -> cfblk2/1
  cfblk12/1 -> cfblk5/1, cfblk3/2
  cfblk9/1 -> cfblk14/1(cfblk1)
  cfblk1/1 -> cfblk13/1
  cfblk7/1 -> cfblk8/2
  cfblk5/1 -> cfblk6/1
  cfblk15/2(cfblk8) -> cfblk7/2, cfblk18/1
  cfblk11/1 -> cfblk14/Action
  cfblk11/2 -> cfblk15/Action
  cfblk4/1 -> cfblk16/1
  cfblk16/1 -> cfblk15/2(cfblk7)
  cfblk15/1(cfblk2) -> cfblk17/1
  cfblk17/1 -> cfblk11/1
  cfblk18/1 -> cfblk3/1

== system sampleModel1/cfblk91/cfblk19 ==
  cfblk1 : Inport
  cfblk6 : Inport  Port=2
  Action Port : ActionPort  ActionPortLabel=else
  cfblk3 : Constant  Value=[165493612.723583]  SampleTime=1
  cfblk4 : Constant  Value=[-930268599.904138]  SampleTime=1
  cfblk5 : Constant  Value=[-184538377.288036]  SampleTime=1
  cfblk2 : Outport
  cfblk7 : Outport  Port=2
  cfblk8 : Outport  Port=3
  wires:
  cfblk1/1 -> cfblk8/1
  cfblk5/1 -> cfblk2/1
  cfblk3/1 -> cfblk7/1

== system sampleModel1/cfblk91/cfblk20 ==
  cfblk1 : Inport
  cfblk11 : Inport  Port=2
  Action Port : ActionPort  ActionPortLabel=if(u1 >= 0)
  cfblk10 : Constant  Value=[113996522.557218]  SampleTime=1
  cfblk12 : Delay
  cfblk3 : Sin  TimeSource=Use external signal  SampleTime=0
  cfblk4 : Signum
  cfblk5 : Squeeze
  cfblk6 : Squeeze
  cfblk7 : Gain  Gain=[-381261515.154502]
  cfblk8 : Constant  Value=[46059596.883986]  SampleTime=1
  cfblk9 : Constant  Value=[663685020.972136]  SampleTime=1
  cfblk2 : Outport
  wires:
  cfblk4/1 -> cfblk6/1
  cfblk11/1 -> cfblk5/1
  cfblk10/1 -> cfblk7/1
  cfblk7/1 -> cfblk2/1
  cfblk9/1 -> cfblk3/1
  cfblk6/1 -> cfblk12/1
  cfblk12/1 -> cfblk4/1

== system sampleModel1/cfblk91/cfblk21 ==
  cfblk1 : Inport
  cfblk10 : Inport  Port=2
  cfblk11 : Inport  Port=3
  Action Port : ActionPort  ActionPortLabel=else
  cfblk3 : simulink/Discrete/Tapped Delay  vinit=0.0  samptime=-1  NumDelays=1  DelayOrder=Oldest  includeCurrent=off
  cfblk4 : Product  Inputs=*
  cfblk5 : Math  Operator=transpose  SaturateOnIntegerOverflow=on
  cfblk6 : Squeeze
  cfblk7 : Product  Inputs=*
  cfblk8 : Constant  Value=[-286992765.745991]  SampleTime=1
  cfblk9 : Constant  Value=[-306636497.490102]  SampleTime=1
  cfblk2 : Outport
  cfblk12 : Outport  Port=2
  cfblk13 : Outport  Port=3
  wires:
  cfblk9/1 -> cfblk12/1
  cfblk10/1 -> cfblk2/1
  cfblk5/1 -> cfblk3/1
  cfblk8/1 -> cfblk7/1
  cfblk7/1 -> cfblk5/1
  cfblk3/1 -> cfblk13/1
  cfblk1/1 -> cfblk4/1
  cfblk4/1 -> cfblk6/1

== system sampleModel1/cfblk91/cfblk9 ==
  cfblk1 : Inport
  cfblk8 : Inport  Port=2
  cfblk10 : Delay
  cfblk3 : DiscreteFilter
  cfblk4 : Product  Inputs=**
  cfblk5 : Product
  cfblk6 : Sum  Inputs=+
  cfblk7 : Constant  Value=[-218290494.547291]  SampleTime=1
  cfblk2 : Outport
  cfblk9 : Outport  Port=2
  wires:
  cfblk4/1 -> cfblk5/1
  cfblk7/1 -> cfblk9/1, cfblk4/2
  cfblk8/1 -> cfblk4/1
  cfblk3/1 -> cfblk2/1
  cfblk5/1 -> cfblk6/1
  cfblk1/1 -> cfblk3/1
  cfblk6/1 -> cfblk10/1
  cfblk10/1 -> cfblk5/2

== system sampleModel1/cfblk92/cfblk17 ==
  cfblk1 : Inport
  cfblk7 : Inport  Port=2
  Action Port : ActionPort  ActionPortLabel=if(u1 >= 0)
  cfblk11 : Subsystem  TreatAsAtomicUnit=on
  cfblk12 : Subsystem  TreatAsAtomicUnit=on
  cfblk13 : Delay
  cfblk14 : Delay
  cfblk15 : Delay
  cfblk3 : Rounding
  cfblk4 : Sum  Inputs=+-
  cfblk5 : Constant  Value=[-196233203.983829]  SampleTime=1
  cfblk6 : If  IfExpression=u1 >= 0  SampleTime=1
  cfblk2 : Outport
  cfblk8 : Outport  Port=2
  cfblk9 : Outport  Port=3
  cfblk10 : Outport  Port=4
  wires:
  cfblk11/2(cfblk11) -> cfblk9/1
  cfblk3/1 -> cfblk11/1(cfblk1)
  cfblk11/3(cfblk12) -> cfblk2/1
  cfblk1/1 -> cfblk10/1
  cfblk7/1 -> cfblk12/1(cfblk1)
  cfblk11/4(cfblk13) -> cfblk8/1
  cfblk5/1 -> cfblk12/2(cfblk10), cfblk4/2
  cfblk12/1(cfblk2) -> cfblk4/1
  cfblk4/1 -> cfblk14/1, cfblk15/1
  cfblk6/1 -> cfblk11/Action
  cfblk6/2 -> cfblk12/Action
  cfblk11/1(cfblk2) -> cfblk13/1
  cfblk13/1 -> cfblk6/1
  cfblk14/1 -> cfblk11/2(cfblk10)
  cfblk15/1 -> cfblk3/1

== system sampleModel1/cfblk92/cfblk18 ==
  cfblk1 : Inport
  cfblk8 : Inport  Port=2
  Action Port : ActionPort  ActionPortLabel=else
  cfblk10 : Subsystem  TreatAsAtomicUnit=on
  cfblk11 : Delay
  cfblk12 : Delay
  cfblk13 : Delay
  cfblk3 : Delay  DelayLengthSource=Input port
      settings: InputPortMap=u0,p1
  cfblk4 : Constant  Value=[-202013154.776741]  SampleTime=1
  cfblk5 : Constant  Value=[-686384224.911209]  SampleTime=1
  cfblk6 : Subsystem
  cfblk7 : If  IfExpression=u1 >= 0  SampleTime=1
  cfblk9 : Subsystem  TreatAsAtomicUnit=on
  cfblk2 : Outport
  wires:
  cfblk8/1 -> cfblk6/1(cfblk1), cfblk10/3(cfblk13)
  cfblk4/1 -> cfblk6/2(cfblk9)
  cfblk5/1 -> cfblk3/1, cfblk10/6(cfblk16)
  cfblk6/1(cfblk2) -> cfblk2/1, cfblk3/2, cfblk11/1
  cfblk10/1(cfblk2) -> cfblk6/3(cfblk10)
  cfblk9/1(cfblk2) -> cfblk10/1(cfblk1)
  cfblk1/1 -> cfblk9/2(cfblk8), cfblk10/5(cfblk15)
  cfblk9/2(cfblk9) -> cfblk10/2(cfblk12)
  cfblk7/1 -> cfblk9/Action
  cfblk7/2 -> cfblk10/Action
  cfblk11/1 -> cfblk10/4(cfblk14)
  cfblk3/1 -> cfblk12/1
  cfblk12/1 -> cfblk7/1
  cfblk10/2(cfblk17) -> cfblk13/1
  cfblk13/1 -> cfblk9/1(cfblk1)

== system sampleModel1/cfblk95/cfblk8 ==
  cfblk1 : Inport
  cfblk9 : Inport  Port=2
  cfblk10 : Inport  Port=3
  cfblk11 : Inport  Port=4
  cfblk3 : UnitDelay  SampleTime=-1  HasFrameUpgradeWarning=on
  cfblk4 : Abs
  cfblk5 : simulink/Math Operations/MinMax Running Resettable  Function=min  vinit=0.0
  cfblk6 : Math  Operator=magnitude^2  SaturateOnIntegerOverflow=on
  cfblk7 : Constant  Value=[845370440.784336]  SampleTime=1
  cfblk8 : Constant  Value=[-52226260.495749]  SampleTime=1
  cfblk2 : Outport
  cfblk12 : Outport  Port=2
  cfblk13 : Outport  Port=3
  cfblk14 : Outport  Port=4
  cfblk15 : Outport  Port=5
  wires:
  cfblk11/1 -> cfblk4/1
  cfblk6/1 -> cfblk15/1
  cfblk5/1 -> cfblk14/1
  cfblk3/1 -> cfblk5/1
  cfblk9/1 -> cfblk3/1
  cfblk7/1 -> cfblk12/1
  cfblk8/1 -> cfblk13/1
  cfblk1/1 -> cfblk5/2
  cfblk4/1 -> cfblk6/1
  cfblk10/1 -> cfblk2/1

== system sampleModel1/cfblk96/cfblk11 ==
  cfblk1 : Inport
  cfblk12 : Inport  Port=2
  cfblk13 : Inport  Port=3
  cfblk14 : Inport  Port=4
  cfblk10 : Subsystem
  cfblk11 : Subsystem
  cfblk3 : Trigonometry
  cfblk4 : ComplexToRealImag
  cfblk5 : Product
  cfblk6 : Reshape
  cfblk7 : Constant  Value=[826364691.801809]  SampleTime=1
  cfblk8 : Constant  Value=[-221614354.014774]  SampleTime=1
  cfblk9 : Constant  Value=[635269719.417462]  SampleTime=1
  cfblk2 : Outport
  cfblk15 : Outport  Port=2
  cfblk16 : Outport  Port=3
  wires:
  cfblk8/1 -> cfblk16/1
  cfblk3/1 -> cfblk4/1
  cfblk9/1 -> cfblk10/1(cfblk1)
  cfblk4/1 -> cfblk11/1(cfblk1)
  cfblk4/2 -> cfblk5/1
  cfblk7/1 -> cfblk15/1
  cfblk1/1 -> cfblk3/1
  cfblk10/1(cfblk2) -> cfblk11/2(cfblk15)
  cfblk14/1 -> cfblk5/2
  cfblk12/1 -> cfblk6/1
  cfblk10/2(cfblk7) -> cfblk2/1

== system sampleModel1/cfblk99/cfblk10 ==
  cfblk1 : Inport
  cfblk10 : Inport  Port=2
  cfblk11 : Inport  Port=3
  cfblk12 : Inport  Port=4
  cfblk13 : Inport  Port=5
  cfblk3 : MinMax  Inputs=2
  cfblk4 : Bias  Bias=[976122571.511085]
  cfblk5 : simulink/Math Operations/MinMax Running Resettable  Function=min  vinit=0.0
  cfblk6 : MinMax  Inputs=2
  cfblk7 : Constant  Value=[-467516241.623746]  SampleTime=1
  cfblk8 : Constant  Value=[-623220916.978346]  SampleTime=1
  cfblk9 : Subsystem
  cfblk2 : Outport
  cfblk14 : Outport  Port=2
  wires:
  cfblk7/1 -> cfblk14/1
  cfblk11/1 -> cfblk5/1
  cfblk3/1 -> cfblk6/1
  cfblk5/1 -> cfblk2/1
  cfblk8/1 -> cfblk9/1(cfblk1)
  cfblk9/1(cfblk2) -> cfblk5/2
  cfblk10/1 -> cfblk9/2(cfblk8)
  cfblk1/1 -> cfblk4/1
  cfblk9/2(cfblk9) -> cfblk3/1
  cfblk9/3(cfblk10) -> cfblk3/2
  cfblk13/1 -> cfblk6/2

== system sampleModel1/cfblk99/cfblk9 ==
  cfblk1 : Inport
  cfblk8 : Inport  Port=2
  cfblk9 : Inport  Port=3
  cfblk10 : Inport  Port=4
  cfblk12 : Subsystem  TreatAsAtomicUnit=on
  cfblk13 : Subsystem  TreatAsAtomicUnit=on
  cfblk14 : Delay
  cfblk15 : Delay
  cfblk3 : Product
  cfblk4 : Constant  Value=[577646330.024922]  SampleTime=1
  cfblk5 : Constant  Value=[657603396.976882]  SampleTime=1
  cfblk6 : Constant  Value=[952293070.454711]  SampleTime=1
  cfblk7 : If  IfExpression=u1 >= 0  SampleTime=1
  cfblk2 : Outport
  cfblk11 : Outport  Port=2
  wires:
  cfblk8/1 -> cfblk13/1(cfblk1)
  cfblk9/1 -> cfblk11/1
  cfblk6/1 -> cfblk2/1
  cfblk1/1 -> cfblk12/1(cfblk1)
  cfblk4/1 -> cfblk12/2(cfblk11)
  cfblk12/1(cfblk2) -> cfblk3/1
  cfblk12/2(cfblk14) -> cfblk3/2
  cfblk5/1 -> cfblk12/3(cfblk12)
  cfblk7/1 -> cfblk12/Action
  cfblk7/2 -> cfblk13/Action
  cfblk3/1 -> cfblk14/1
  cfblk14/1 -> cfblk7/1
  cfblk13/1(cfblk2) -> cfblk15/1
  cfblk15/1 -> cfblk12/4(cfblk13)

== system sampleModel1/cfblk103/cfblk5/cfblk18 ==
  cfblk1 : Inport
  cfblk6 : Inport  Port=2
  cfblk7 : Inport  Port=3
  Action Port : ActionPort  ActionPortLabel=if(u1 >= 0)
  cfblk3 : Math  Operator=10^u  SaturateOnIntegerOverflow=on
  cfblk4 : UnaryMinus
  cfblk5 : Constant  Value=[331654320.089606]  SampleTime=1
  cfblk2 : Outport
  wires:
  cfblk1/1 -> cfblk3/1
  cfblk3/1 -> cfblk2/1
  cfblk5/1 -> cfblk4/1

== system sampleModel1/cfblk103/cfblk5/cfblk19 ==
  cfblk1 : Inport
  cfblk13 : Inport  Port=2
  cfblk14 : Inport  Port=3
  cfblk15 : Inport  Port=4
  cfblk16 : Inport  Port=5
  Action Port : ActionPort  ActionPortLabel=else
  cfblk10 : Constant  Value=[-943441098.208414]  SampleTime=1
  cfblk11 : Constant  Value=[592212471.885680]  SampleTime=1
  cfblk12 : Subsystem
  cfblk3 : Assignment  DiagnosticForDimensions=Warning  IndexOptions=Index vector (dialog)  Indices=1  OutputSizes=1
  cfblk4 : PermuteDimensions
  cfblk5 : Sqrt  Operator=rSqrt  AlgorithmType=Newton-Raphson  SaturateOnIntegerOverflow=on
  cfblk6 : ComplexToRealImag
  cfblk7 : Constant  Value=[-896116037.263308]  SampleTime=1
  cfblk8 : Constant  Value=[684689403.657546]  SampleTime=1
  cfblk9 : Constant  Value=[-121950224.681572]  SampleTime=1
  cfblk2 : Outport
  wires:
  cfblk13/1 -> cfblk4/1
  cfblk7/1 -> cfblk6/1
  cfblk8/1 -> cfblk3/1
  cfblk9/1 -> cfblk12/1(cfblk1)
  cfblk10/1 -> cfblk3/2
  cfblk3/1 -> cfblk12/2(cfblk5)
  cfblk1/1 -> cfblk12/3(cfblk6)
  cfblk15/1 -> cfblk2/1
  cfblk12/1(cfblk2) -> cfblk5/1

== system sampleModel1/cfblk103/cfblk5/cfblk20 ==
  cfblk1 : Inport
  cfblk11 : Inport  Port=2
  Action Port : ActionPort  ActionPortLabel=if(u1 >= 0)
  cfblk10 : If  IfExpression=u1 >= 0  SampleTime=1
  cfblk12 : Subsystem  TreatAsAtomicUnit=on
  cfblk13 : Subsystem  TreatAsAtomicUnit=on
  cfblk{14..19} (6 alike) : Delay
  cfblk3 : simulink/Discrete/Difference  ICPrevInput=0.0  OutMin=[]  OutMax=[]  OutDataTypeStr=Inherit: Inherit via back propagation  OutDataType=fixdt(1, 16)  OutScaling=2^-10  DoSatur=off
  cfblk4 : simulink/Discrete/Transfer Fcn First Order  PoleZ=0.95  ICPrevOutput=0.0  DoSatur=off
  cfblk5 : Bias  Bias=[352460180.564506]
  cfblk6 : Constant  Value=[-248483657.565017]  SampleTime=1
  cfblk7 : Constant  Value=[-416046498.027941]  SampleTime=1
  cfblk8 : Constant  Value=[345301028.854859]  SampleTime=1
  cfblk9 : Subsystem
  cfblk2 : Outport
  wires:
  cfblk7/1 -> cfblk2/1, cfblk12/5(cfblk13)
  cfblk11/1 -> cfblk9/2(cfblk13)
  cfblk6/1 -> cfblk5/1
  cfblk8/1 -> cfblk3/1
  cfblk5/1 -> cfblk13/1(cfblk1)
  cfblk12/1(cfblk2) -> cfblk9/3(cfblk14)
  cfblk12/2(cfblk15) -> cfblk4/1
  cfblk3/1 -> cfblk13/2(cfblk10), cfblk12/6(cfblk14)
  cfblk1/1 -> cfblk12/2(cfblk10)
  cfblk10/1 -> cfblk12/Action
  cfblk10/2 -> cfblk13/Action
  cfblk9/1(cfblk2) -> cfblk14/1
  cfblk14/1 -> cfblk13/3(cfblk11)
  cfblk13/1(cfblk2) -> cfblk15/1
  cfblk15/1 -> cfblk9/1(cfblk1)
  cfblk13/2(cfblk12) -> cfblk16/1
  cfblk16/1 -> cfblk10/1
  cfblk9/2(cfblk15) -> cfblk17/1
  cfblk17/1 -> cfblk12/3(cfblk11)
  cfblk9/3(cfblk16) -> cfblk18/1
  cfblk18/1 -> cfblk12/4(cfblk12)
  cfblk4/1 -> cfblk19/1
  cfblk19/1 -> cfblk12/1(cfblk1)

== system sampleModel1/cfblk103/cfblk5/cfblk21 ==
  cfblk1 : Inport
  Action Port : ActionPort  ActionPortLabel=else
  cfblk10 : Product
  cfblk11 : Sin  TimeSource=Use external signal  SampleTime=0
  cfblk12 : Constant  Value=[678283610.279772]  SampleTime=1
  cfblk13 : Subsystem
  cfblk16 : Delay
  cfblk3 : DiscreteIntegrator  SampleTime=-1  ICPrevOutput=DiscIntNeverNeededParam  ICPrevScaledInput=DiscIntNeverNeededParam
  cfblk4 : simulink/Discrete/Difference  ICPrevInput=0.0  OutMin=[]  OutMax=[]  OutDataTypeStr=Inherit: Inherit via back propagation  OutDataType=fixdt(1, 16)  OutScaling=2^-10  DoSatur=off
  cfblk5 : DiscreteZeroPole  Poles=[0 0.5]  Gain=1  SampleTime=-1
  cfblk6 : Sum  Inputs=+-
  cfblk7 : Abs
  cfblk8 : Sqrt  Operator=rSqrt  AlgorithmType=Newton-Raphson  SaturateOnIntegerOverflow=on
  cfblk9 : Polyval  Coefs=[ +2.081618890e-019, -1.441693666e-014, +4.719686976e-010, -8.536869453e-006, +1.621573104e-001, -8.087801117e+001 ]
  cfblk2 : Outport
  cfblk14 : Outport  Port=2
  cfblk15 : Outport  Port=3
  wires:
  cfblk9/1 -> cfblk6/1
  cfblk12/1 -> cfblk7/1
  cfblk10/1 -> cfblk11/1
  cfblk3/1 -> cfblk13/1(cfblk1)
  cfblk7/1 -> cfblk2/1, cfblk6/2
  cfblk4/1 -> cfblk15/1
  cfblk6/1 -> cfblk8/1, cfblk10/2
  cfblk11/1 -> cfblk4/1
  cfblk1/1 -> cfblk14/1, cfblk10/1
  cfblk8/1 -> cfblk5/1
  cfblk13/1(cfblk2) -> cfblk9/1
  cfblk5/1 -> cfblk16/1
  cfblk16/1 -> cfblk3/1

== system sampleModel1/cfblk103/cfblk5/cfblk9 ==
  cfblk1 : Inport
  cfblk14 : Inport  Port=2
  cfblk15 : Inport  Port=3
  cfblk16 : Inport  Port=4
  cfblk10 : Constant  Value=[486427548.401634]  SampleTime=1
  cfblk11 : Constant  Value=[188365825.939887]  SampleTime=1
  cfblk12 : Constant  Value=[135705318.575576]  SampleTime=1
  cfblk13 : Subsystem
  cfblk17 : Delay
  cfblk3 : DiscreteStateSpace  SampleTime=-1
  cfblk4 : simulink/Discrete/Transfer Fcn Lead or Lag  PoleZ=0.95  ZeroZ=0.75  ICPrevOutput=0.0  ICPrevInput=0.0  DoSatur=off
      settings: SourceProductBaseCode=SL
  cfblk5 : ComplexToMagnitudeAngle
  cfblk6 : Sin  TimeSource=Use external signal  SampleTime=0
  cfblk7 : Signum
  cfblk8 : Sum  Inputs=-+
  cfblk9 : Polyval  Coefs=[ +2.081618890e-019, -1.441693666e-014, +4.719686976e-010, -8.536869453e-006, +1.621573104e-001, -8.087801117e+001 ]
  cfblk2 : Outport
  wires:
  cfblk5/1 -> cfblk8/1
  cfblk7/1 -> cfblk4/1
  cfblk13/1(cfblk2) -> cfblk6/1
  cfblk8/1 -> cfblk7/1
  cfblk16/1 -> cfblk13/1(cfblk1)
  cfblk3/1 -> cfblk8/2
  cfblk5/2 -> cfblk9/1
  cfblk11/1 -> cfblk3/1
  cfblk13/2(cfblk6) -> cfblk2/1
  cfblk9/1 -> cfblk17/1
  cfblk17/1 -> cfblk5/1

== system sampleModel1/cfblk104/cfblk18/cfblk10 ==
  cfblk1 : Inport
  Action Port : ActionPort  ActionPortLabel=else
  cfblk3 : pid_lib/PID Controller  Controller=PID  Form=Parallel  TimeDomain=Discrete-time  UseExternalTs=off  SampleTime=-1  IntegratorMethod=Forward Euler  FilterMethod=Forward Euler  ControllerParametersSource=internal  P=1  I=1  D=0  UseFilter=on  N=100  TunerSelectOption=Transfer Function Based (PID Tuner App)  InitialConditionSource=internal  InitialConditionForIntegrator=0  InitialConditionForFilter=0  DifferentiatorICPrevScaledInput=0  ExternalReset=none  TrackingMode=off  Kt=1  LimitOutput=off  SatLimitsSource=internal  UpperSaturationLimit=inf  LowerSaturationLimit=-inf  LinearizeAsGain=off  AntiWindupMode=none  Kb=1  POutMin=[]  POutMax=[]  IOutMin=[]  IOutMax=[]  DOutMin=[]  DOutMax=[]  NOutMin=[]  NOutMax=[]  SumOutMin=[]  SumOutMax=[]  SaturationOutMin=[]  SaturationOutMax=[]  PParamMin=[]  PParamMax=[]  IParamMin=[]  IParamMax=[]  DParamMin=[]  DParamMax=[]  NParamMin=[]  NParamMax=[]  KbParamMin=[]  KbParamMax=[]  KtParamMin=[]  KtParamMax=[]  KbOutMin=[]  KbOutMax=[]  KtOutMin=[]  KtOutMax=[]  IntegratorOutMin=[]  IntegratorOutMax=[]  FilterOutMin=[]  FilterOutMax=[]  SumI1OutMin=[]  SumI1OutMax=[]  SumI2OutMin=[]  SumI2OutMax=[]  SumI3OutMin=[]  SumI3OutMax=[]  SumI4OutMin=[]  SumI4OutMax=[]  SumDOutMin=[]  SumDOutMax=[]  DifferentiatorOutMin=[]  DifferentiatorOutMax=[]  FilterDiffOutCoefMin=[]  FilterDiffOutCoefMax=[]  ReciprocalOutMin=[]  ReciprocalOutMax=[]  SumDenOutMin=[]  SumDenOutMax=[]  SumNumOutMin=[]  SumNumOutMax=[]  DivideOutMin=[]  DivideOutMax=[]  UdiffTsProdOutMin=[]  UdiffTsProdOutMax=[]  NTsProdOutMin=[]  NTsProdOutMax=[]  UintegralTsProdOutMin=[]  UintegralTsProdOutMax=[]  UngainTsProdOutMin=[]  UngainTsProdOutMax=[]  IntegratorContinuousStateAttributes=''  IntegratorStateMustResolveToSignalObject=off  IntegratorRTWStateStorageClass=Auto  FilterContinuousStateAttributes=''  FilterStateMustResolveToSignalObject=off  FilterRTWStateStorageClass=Auto  ParallelPVariant=InternalParameters  IdealPVariant=Disabled  IVariant=InternalParameters  DVariant=InternalParameters  IntegratorVariant=Discrete  SatVariant=Disabled  AWVariant=Passthrough  PCopyVariant=Disabled  TRVariant=Disabled  FdbkBlocksVariant=Forward  IdealPFdbkVariant=Disabled  SatFdbkVariant=Disabled  DerivativeFilterVariant=ForwardEulerFilter  NVariant=InternalParameters  NCopyVariant=Disabled  FilterICVariant=InternalICsFilter  IntegratorICVariant=InternalICs  ExternalResetVariant=Disabled  TRSumVariant=Passthrough  SumFdbkVariant=Disabled  SumVariant=Sum_PID  TsampFilterVariant=InternalTs  TsampNgainVariant=Passthrough  TsampIntegralVariant=Passthrough  ExternalSaturationOutDataTypeStr=Inherit: Same as second input
  cfblk4 : Constant  Value=[768904473.809565]  SampleTime=1
  cfblk5 : Constant  Value=[818099683.885603]  SampleTime=1
  cfblk2 : Outport
  cfblk6 : Outport  Port=2
  cfblk7 : Outport  Port=3
  wires:
  cfblk4/1 -> cfblk3/1
  cfblk5/1 -> cfblk6/1
  cfblk1/1 -> cfblk2/1
  cfblk3/1 -> cfblk7/1

== system sampleModel1/cfblk104/cfblk18/cfblk9 ==
  cfblk1 : Inport
  cfblk9 : Inport  Port=2
  cfblk10 : Inport  Port=3
  Action Port : ActionPort  ActionPortLabel=if(u1 >= 0)
  cfblk11 : Delay
  cfblk12 : Delay
  cfblk3 : simulink/Discrete/Difference  ICPrevInput=0.0  OutMin=[]  OutMax=[]  OutDataTypeStr=Inherit: Inherit via back propagation  OutDataType=fixdt(1, 16)  OutScaling=2^-10  DoSatur=off
  cfblk4 : Sin  TimeSource=Use external signal  SampleTime=0
  cfblk5 : Polyval  Coefs=[ +2.081618890e-019, -1.441693666e-014, +4.719686976e-010, -8.536869453e-006, +1.621573104e-001, -8.087801117e+001 ]
  cfblk6 : Trigonometry
  cfblk7 : Constant  Value=[-246879146.014232]  SampleTime=1
  cfblk8 : Subsystem
  cfblk2 : Outport
  wires:
  cfblk8/1(cfblk2) -> cfblk5/1
  cfblk6/1 -> cfblk8/1(cfblk1)
  cfblk4/1 -> cfblk6/1
  cfblk10/1 -> cfblk4/1
  cfblk7/1 -> cfblk2/1
  cfblk3/1 -> cfblk8/3(cfblk14)
  cfblk9/1 -> cfblk8/4(cfblk15)
  cfblk5/1 -> cfblk11/1
  cfblk11/1 -> cfblk8/2(cfblk13)
  cfblk8/2(cfblk16) -> cfblk12/1
  cfblk12/1 -> cfblk3/1
